simulink model "simpleTest"  (R2023a)
settings: Solver=FixedStepAuto  StartTime=0.0  StopTime=endTime  FixedStep=stepSize  RelTol=1e-3  AbsTol=1e-3  EnableMultiTasking=on
undefined symbols (not defined in the file or in its folder): arm, DiscIntNeverNeededParam, jointControlData, X, Y, Z
libraries: nesl_utility x44, sm_lib x18
(part 2 of 2)

== matlab function simpleTest/MATLAB Function3 ==
  data: time input; Hom1 input; geometry1 input; momentum output; massProperties1 input; nLink1 input; Hom2 input; geometry2 input; massProperties2 input; nLink2 input; base_state input; arm1_state input; arm2_state input; desired_rates output
function [momentum,desired_rates] = computeMomentum(time,Hom1,geometry1,massProperties1,nLink1,Hom2,geometry2,massProperties2,nLink2,base_state,arm1_state,arm2_state)

% Extract variables from structure for convenience
rBase1 = geometry1.rBase;
RLbase1 = geometry1.RLbase;
RL1 = geometry1.RL;
rVec1  = geometry1.rVec;
rVec01 = geometry1.rVec0;
pVec1  = geometry1.pVec;
kVec1  = geometry1.kVec;
massVec1 = massProperties1.massVec;
inertiaMatBase1 = massProperties1.inertiaMatBase;
linkInertia1 = massProperties1.linkInertia;

rBase2 = geometry2.rBase;
RLbase2 = geometry2.RLbase;
RL2 = geometry2.RL;
rVec2  = geometry2.rVec;
rVec02 = geometry2.rVec0;
pVec2  = geometry2.pVec;
kVec2  = geometry2.kVec;
massVec2 = massProperties2.massVec;
linkInertia2 = massProperties2.linkInertia;

% Compute the vector from base to system center of mass
roc = base_state(1:3)' - rBase1(:)';
rocSkew = skewMat(roc);

% Mass of base
mt = massVec1(1);

% Form the inertia matrix of the base - manipulator system
HsBase = RLbase1*inertiaMatBase1*RLbase1';

Hs1 = zeros(3,3);
Hs2 = zeros(3,3);

for i = 1:nLink1
    rSkew = skewMat(rVec01(i,:));
    Hs1 = squeeze(linkInertia1(i,:,:)) - massVec1(i+1)*rSkew*rSkew;  % Ref 1, Eq. 29 
    mt = mt + massVec1(i+1);
end
for i = 1:nLink2
    rSkew = skewMat(rVec02(i,:));
    Hs2 = squeeze(linkInertia2(i,:,:)) - massVec2(i+1)*rSkew*rSkew;  % Ref 1, Eq. 29 
    mt = mt + massVec2(i+1);
end

Hs = HsBase + Hs1 + Hs2;

% Form the base-spacecraft inertia matrix
Ho = [mt*eye(3,3) -mt*rocSkew; mt*rocSkew Hs];           % Ref 1, Eq. 28

% Compute linear and angular momentum     
momentum = Ho*base_state(7:end) + Hom1*arm1_state + Hom2*arm2_state;

% Compute desired rates for arm 2
desired_rates = -1*pinv(Hom2)*(1*Ho*base_state(7:end) + Hom1*arm1_state);
% desired_rates = -1*pinv(Hom2(4:6))*(-1*Ho(4:6)*base_state(10:end) + Hom1(4:6)*arm1_state);
desired_rates = -1*pinv(Hom2(4:6))*(Hom1(4:6)*arm1_state);
% desired_rates = -1*pinv(Hom2)*(Hom1*arm1_state);
